simulink model "isop_dual_active_bridge"  (Simulink 7.3)
settings: Solver=ode45  StartTime=0.0  StopTime=0.05  RelTol=1e-3
InitFcn:
  | % Processor selection for I/O assignment
  | % The chosen Target in the Coder Options window must match the selected MCU.
  | % Set the variable 'type_evm' to the following strings to choose a specific target:
  | 
  |   type_evm = 'TI28069';        % TI28069 Piccolo Launchpad
  | % type_evm = 'TI28379LP';  % TI28379D Delfino Launchpad
  | % type_evm = 'TI28379CC';  % TI28379D Delfino Controlcard
  | % type_evm = 'TI28388D';    % TI28388D Controlcard
  | 
  | % Configure I/O based on processor
  | switch (type_evm)
  | 	case 'TI28069'
  | 	% Configuration for TI28069 Launchpad
  | 	% On the Plant side
  | 		AO_RTBox_VLV = 0;
  | 		AO_RTBox_VHV1 = 1;
  |       AO_RTBox_ILV1 = 2;
  | 		AO_RTBox_VHV2 = 3;
  | 		AO_RTBox_ILV2 = 4;
  | 		AO_RTBox_VC1 = 5;
  | 		AO_RTBox_VC2 = 6;
  | 		PWM_capture_1_channels = [0 1 2 3];
  | 		PWM_capture_2_channels = [16 17 18 19];
  | 
  | 		DI_RTBox_Eni = 29;			% Global enable emulated by sliding switch 29
  | 		DO_RTBox_Eno = 4;			% Global enable DO
  | 		DI_RTBox_Tzi = 28;			% TZ1 DI emulated with sliding switch
  | 		DO_RTBox_Tzo = 2;			% TZ1 DO
  | 		DI_RTBox_Power = 22;			% Powerstage enable DI
  | 
  | 		AO_Factor = 1;
  | 		AO_Vmax = 3.3;
  | 
  | 	% On the MCU side
  | 		DSP_ADC_channels = [7 1+8 2 2+8 0 0+8 1];
  | 		DO_DSP_LED = 34;
  | 		DI_DSP_En = 13;				% Global enable DI
  | 		TZ_DSP_Tz1 = 12;				% TZ1 DI
  | 		PWR_DSP_GPIO = 27;			% Powerstage enable DO
  | 		SCI_DSP = [28, 29];
  | 		ADC_Vmax = 3.3;
  | 
  | 	case 'TI28379LP'
  | 	% Configuration for TI28379D Launchpad
  | 	% On the Plant side
  | 		AO_RTBox_VLV = 0;
  | 		AO_RTBox_VHV1 = 3;
  |       AO_RTBox_ILV1 = 7;
  | 		AO_RTBox_VHV2 = 11;
  | 		AO_RTBox_ILV2 = 14;
  | 		AO_RTBox_VC1 = 15;
  | 		AO_RTBox_VC2 = 8;
  | 		PWM_capture_1_channels = [0 1 2 3];
  | 		PWM_capture_2_channels = [16 17 18 19];
  | 
  | 		DI_RTBox_Eni = 29;
  | 		DO_RTBox_Eno = 6;
  | 		DI_RTBox_Tzi = 28;
  | 		DO_RTBox_Tzo = 7;
  | 		DI_RTBox_Power = 22;
  | 
  | 		AO_Factor = 1;
  | 		AO_Vmax = 3.3;
  | 
  | 	% On the MCU side
  |       DSP_ADC_channels = [14 3 0 5 4 1 15];
  | 		DO_DSP_LED = 34;
  | 		DI_DSP_En = 124;
  | 		TZ_DSP_Tz1 = 125;
  | 		PWR_DSP_GPIO = 66;
  | 		SCI_DSP = [43, 42];
  | 		ADC_Vmax = 3.3;
  | 
  | 	case 'TI28379CC'
  | 	% Configuration for TI28379D Controlcard
  | 	% On the Plant side
  | 	   AO_RTBox_VLV = 15;
  | 		AO_RTBox_VHV1 = 13;
  |       AO_RTBox_ILV1 = 11;
  | 		AO_RTBox_VHV2 = 9;
  | 		AO_RTBox_ILV2 = 7;
  | 		AO_RTBox_VC1 = 5;
  | 		AO_RTBox_VC2 = 3;
  | 		PWM_capture_1_channels = [0 1 2 3];
  | 		PWM_capture_2_channels = [6 7 8 9];
  | 
  | 		DI_RTBox_Eni = 29;
  | 		DO_RTBox_Eno = 21;
  | 		DI_RTBox_Tzi = 28;
  | 		DO_RTBox_Tzo = 20;
  | 		DI_RTBox_Power = 14;
  | 
  | 		AO_Factor = 1.54; % breakout board scaling 6.8k/4.42k
  | 		AO_Vmax = 5.0;
  | 
  | 		% On the MCU side
  |       DSP_ADC_channels = [0 1 2 3 4 5 14];
  | 		DO_DSP_LED = 34;
  | 		DI_DSP_En = 40;
  | 		TZ_DSP_Tz1 = 41;
  | 		PWR_DSP_GPIO = 39;
  | 		SCI_DSP = [28, 29];
  | 		ADC_Vmax = 3.0;
  | 
  | 
  | 	case 'TI28388D'
  | 	% Configuration for TI28388D Controlcard
  | 	% On the Plant side
  | 	   AO_RTBox_VLV = 15;
  | 		AO_RTBox_VHV1 = 13;
  |       AO_RTBox_ILV1 = 11;
  | 		AO_RTBox_VHV2 = 9;
  | 		AO_RTBox_ILV2 = 7;
  | 		AO_RTBox_VC1 = 5;
  | 		AO_RTBox_VC2 = 3;
  | 		PWM_capture_1_channels = [0 1 2 3];
  | 		PWM_capture_2_channels = [6 7 8 9];
  | 
  | 		DI_RTBox_Eni = 29;
  | 		DO_RTBox_Eno = 21;
  | 		DI_RTBox_Tzi = 28;
  | 		DO_RTBox_Tzo = 20;
  | 		DI_RTBox_Power = 14;
  | 
  | 		AO_Factor = 1.54; % breakout board scaling 6.8k/4.42k
  | 		AO_Vmax = 5.0;
  | 
  | 		% On the MCU side
  |       DSP_ADC_channels = [0 1 2 3 4 5 14];
  | 		DO_DSP_LED = 34;
  | 		DI_DSP_En = 40;
  | 		TZ_DSP_Tz1 = 41;
  | 		PWR_DSP_GPIO = 39;
  | 		SCI_DSP = [28, 29];
  | 		ADC_Vmax = 3.0;
  | 
  | 	otherwise
  | 	error('Unknown evaluation module selection, please choose either ''TI28069'', ''TI28379LP'', ''TI28379CC'' or ''TI28388D''.')
  | end
  | 
  | 
  | %% DAB Inductor Design
  | Vlv = 120;								% Battery-side voltage (V)
  | Vhv = 350;								% DC Grid-side voltage (V)
  | n = Vhv/Vlv;							          % Transformer turns ratio (p.u.)
  | Pnom = 10e3;							% Nominal DAB power (W)
  | Clv = 1e-3;								% Low-voltage side capacitance (F)
  | Chv = 1e-3;
  | Llv = 2e-5;								% Low-voltage side inductor (H)
  | Rllv = 0.1;								% Winding resistance of low-voltage side inductor (Ohms)
  | fsw = 15e3;								% Switching frequency (Hz)
  | Rtot = 0.1;								% Transformer winding resistance (Ohms)
  | Ltot = n*Vhv*Vlv/(8*fsw*Pnom)		                              % Total longitudal inductor (H)
  | 
  | %% General Parameters
  | Tdisc.Plant = 3.5e-6;				                    % Discretization step size for DAB plant (s)
  | Tdisc.Control = 1/fsw;				                    % Discretization step size for Controller execution
  | 
  | fc = 1e3; 								% Cut-off frequency of the AAF
  | 
  | % Limits for current reference
  | SatIUp = Pnom/Vlv;					          % Upper saturation limit
  | SatILow = -Pnom/Vlv;					          % Lower saturation limit
  | 
  | Inom = 0.99*SatIUp;					          % Nominal current (A)
  | 
  | % Controller
  | KpCurrent = 0.5;
  | KiCurrent = 225;
  | 
  | KpVoltage = 1.0;
  | 
  | % Voltage balancing controller
  | KpBalance = 10;
  | 
  | %% Analog In\Out scaling
  | 
  | I_LV_max = 400;
  | I_LV_range = ADC_Vmax;
  | I_LV_scale =I_LV_range/2/I_LV_max;
  | I_LV_offset = ADC_Vmax/2;
  | 
  | V_LV_max = Vlv*1.25;
  | V_LV_range = ADC_Vmax;
  | V_LV_scale = V_LV_range/V_LV_max;
  | V_LV_offset = 0;
  | 
  | V_HV_max = Vhv*1.25;
  | V_HV_range = ADC_Vmax;
  | V_HV_scale = V_HV_range/V_HV_max;
  | V_HV_offset = 0;
  | 
  | V_C_max = Vhv*1.25;
  | V_C_range = ADC_Vmax;
  | V_C_scale = V_C_range/2/V_C_max;
  | V_C_offset = V_C_range/2;
  | 
  | % DSP Analog In Configuration
  | DSP_ADC_scale = [1/V_LV_scale 1/V_HV_scale 1/I_LV_scale 1/V_HV_scale 1/I_LV_scale 1/V_C_scale 1/V_C_scale];
  | DSP_ADC_offset = [0 0 -I_LV_offset/I_LV_scale 0 -I_LV_offset/I_LV_scale -V_C_offset/V_C_scale -V_C_offset/V_C_scale];
undefined symbols (not defined in the file): plecs
settings Model: Creator=kris  LastModifiedBy=manaswini  ExtModeTrigMode=oneshot  ExtModeArmWhenConnect=off  ExtModeAutoUpdateStatusClock=off
settings DataIOCC: LimitDataPoints=off  ReturnWorkspaceOutputs=off  SignalLoggingName=sigsOut
settings OptimizationCC: BooleanDataType=off  ExpressionDepthLimit=128  InitFltsAndDblsToZero=on
settings DebuggingCC: SaveWithParameterizedLinksMsg=none  SignalResolutionControl=TryResolveAllWithWarning  SolverPrmCheckMsg=none  MultiTaskDSMMsg=warning  MultiTaskCondExecSysMsg=none  FcnCallInpInsideContextMsg=Enable All  StrictBusMsg=ErrorLevel1
settings HardwareCC: TargetHWDeviceType=32-bit Generic  TargetUnknown=on  ProdEqTarget=off
settings RTWCC: IncludeERTFirstTime=on
settings CodeAppCC: CustomSymbolStrType=$N$R$M_T
settings GRTTargetCC: TargetFcnLib=ansi_tfl_tmw.mat  TargetFunctionLibrary=C89/C90 (ANSI)  ModelReferenceCompliant=off

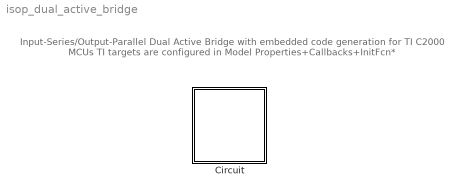
== system isop_dual_active_bridge ==
  note: Input-Series/Output-Parallel Dual Active Bridge
      | with embedded code generation for TI C2000 MCUs
      | TI targets are configured in Model Properties+Callbacks+InitFcn*
  Circuit : Subsystem  LoadFcn=plecs('sl', 200);  InitFcn=plecs('sl', 214);  StartFcn=plecs('sl', 208);  StopFcn=plecs('sl', 209);  ClipboardFcn=plecs('sl', 212, 42);  mask(PlecsCircuit){PLECSData=<binary blob, 24900 chars, not shown>}
      mask prompts: PLECSData "PLECS Data (Do not delete or modify!)"
      mask help: Drag this block into a Simulink model to create a new electrical circuit.
      mask init:
      | % PLACE CUSTOM INITIALIZATIONS ABOVE
      | % DO NOT REMOVE
      | plecs('sl', 215);
      | % DO NOT REMOVE
      settings: CopyFcn=plecs('sl', 203);  DeleteFcn=plecs('sl', 205);  UndoDeleteFcn=plecs('sl', 206);  PreSaveFcn=plecs('sl', 211);  PostSaveFcn=plecs('sl', 201);  NameChangeFcn=plecs('sl', 210);  DestroyFcn=plecs('sl', 207);  PreCopyFcn=plecs('sl', 216);  OpenFcn=plecs('sl', 202);  ErrorFcn=plerrorfcn
      mask Display: disp('PLECS\nCircuit')

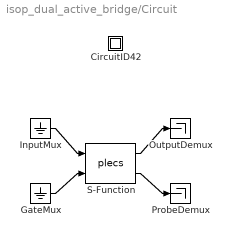
== system isop_dual_active_bridge/Circuit ==
  " CircuitID42 " : Subsystem
  " GateMux " : Ground
  " InputMux " : Ground
  " OutputDemux " : Terminator
  " ProbeDemux " : Terminator
  " S-Function " : S-Function  FunctionName=plecs  EnableBusSupport=off
  wires:
  " InputMux "/1 -> " S-Function "/1
  " GateMux "/1 -> " S-Function "/2
  " S-Function "/1 -> " OutputDemux "/1
  " S-Function "/2 -> " ProbeDemux "/1

== system isop_dual_active_bridge/Circuit/ CircuitID42  ==
